simulink model "hover_test"  (R2017b)
settings: Solver=VariableStepAuto  StartTime=0.0  StopTime=30  RelTol=1e-3
libraries: NLGCToolbox x2
settings Model: Creator=hoang  LastModifiedBy=hoang

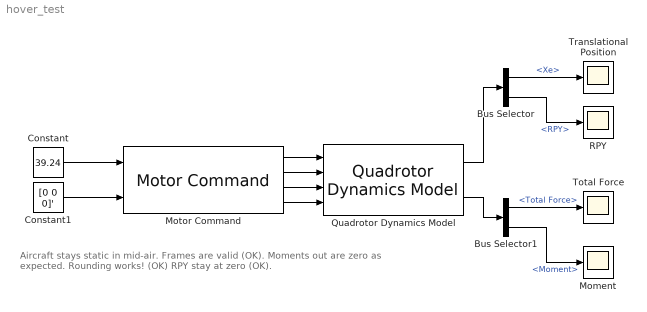
== system hover_test ==
  note: Aircraft stays static in mid-air.
      | Frames are valid (OK).
      | Moments out are zero as expected. Rounding works! (OK)
      | RPY stay at zero (OK).
  Bus Selector : BusSelector  OutputSignals=Xe,RPY
  Bus Selector1 : BusSelector  OutputSignals=Total Force,Moment
  Constant : Constant  Value=39.24
  Constant1 : Constant  Value=[0 0 0]'
  Moment : Scope
  Motor Command : NLGCToolbox/Motor Command  quadrotor=quad
      settings: SourceProductName=Thinh - NLGC for Quadrotor
  Quadrotor Dynamics Model : NLGCToolbox/Quadrotor Dynamics Model  xinit=[0 0 -4]  quadrotor=quad
      settings: SourceProductName=Thinh - NLGC for Quadrotor
  RPY : Scope
  Total Force : Scope
  Translational Position : Scope
  wires:
  Motor Command/1 -> Quadrotor Dynamics Model/1
  Motor Command/2 -> Quadrotor Dynamics Model/2
  Motor Command/3 -> Quadrotor Dynamics Model/3
  Motor Command/4 -> Quadrotor Dynamics Model/4
  Constant/1 -> Motor Command/1
  Constant1/1 -> Motor Command/2
  Quadrotor Dynamics Model/1 -> Bus Selector/1
  Bus Selector/1 -> Translational Position/1  "<Xe>"
  Bus Selector/2 -> RPY/1  "<RPY>"
  Quadrotor Dynamics Model/2 -> Bus Selector1/1
  Bus Selector1/1 -> Total Force/1  "<Total Force>"
  Bus Selector1/2 -> Moment/1  "<Moment>"
